simulink model "simulation"  (R2020a)
settings: Solver=VariableStepAuto  StartTime=0.0  StopTime=55  RelTol=1e-3
values from neighbouring files (symbols this model uses):
  gates = [zeros(36,1);zeros(3*length(cars)/18,1)]    [init.m]
  isReroute = 0    [init.m]
  J = 10000000    [init.m]
  rule = 1    [init.m]
  sequences = cars    [init.m]
  T = 10000000    [init.m]
  threshold = 200    [init.m]
  x0 = [reshape(areas,45,1);cars]    [init.m]
libraries: simulink x9
settings Model: Creator=Admin  LastModifiedBy=Admin

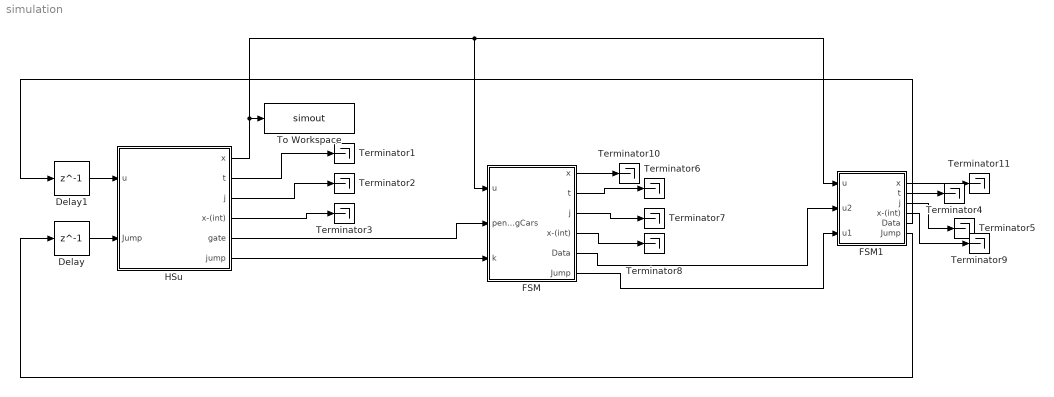
== system simulation ==
  Delay : Delay  DelayLength=1  InitialCondition=0
  Delay1 : Delay  DelayLength=1  InitialCondition=0
  FSM : Subsystem  LoadFcn=set_param(gcb,'LinkStatus','none')
      settings: CopyFcn=|
      | set_param(gcb,'LinkStatus','none'),
      | set_param(gcs, 'MaxStep', 'MaxStep', 'RelTol', 'RelTol','Stop time', 'T')
      mask Display:
      | image(imread('FSM.jpg'))
      | %plot([5 20 20 5 5],[5 5 20 20 5])
      | %text(8,13,'HyEq_mdl')
      | port_label('output', 1, 'x')
      | port_label('output', 2, 't')
      | port_label('output', 3, 'j')
      | port_label('output', 4, 'x-(int)')
      | port_label('input', 1, 'u')
  FSM1 : Subsystem  LoadFcn=set_param(gcb,'LinkStatus','none')
      settings: CopyFcn=|
      | set_param(gcb,'LinkStatus','none'),
      | set_param(gcs, 'MaxStep', 'MaxStep', 'RelTol', 'RelTol','Stop time', 'T')
      mask Display:
      | image(imread('FSM.jpg'))
      | %plot([5 20 20 5 5],[5 5 20 20 5])
      | %text(8,13,'HyEq_mdl')
      | port_label('output', 1, 'x')
      | port_label('output', 2, 't')
      | port_label('output', 3, 'j')
      | port_label('output', 4, 'x-(int)')
      | port_label('input', 1, 'u')
  HSu : Subsystem  LoadFcn=set_param(gcb,'LinkStatus','none')
      settings: CopyFcn=|
      | set_param(gcb,'LinkStatus','none'),
      | set_param(gcs, 'MaxStep', 'MaxStep', 'RelTol', 'RelTol','Stop time', 'T')
      mask Display:
      | image(imread('Cplant.jpg'))
      | %plot([5 20 20 5 5],[5 5 20 20 5])
      | %text(8,13,'HyEq_mdl')
      | port_label('output', 1, 'x')
      | port_label('output', 2, 't')
      | port_label('output', 3, 'j')
      | port_label('output', 4, 'x-(int)')
      | port_label('input', 1, 'u')
  Terminator{1..11} (11 alike) : Terminator
  To Workspace : ToWorkspace  VariableName=simout  SaveFormat=Timeseries  SampleTime=-1
  wires:
  FSM/2(t) -> Terminator6/1
  FSM/3(j) -> Terminator7/1
  FSM/4(x-(int)) -> Terminator8/1
  HSu/2(t) -> Terminator1/1
  HSu/3(j) -> Terminator2/1
  HSu/4(x-(int)) -> Terminator3/1
  FSM1/4(x-(int)) -> Terminator9/1
  FSM1/3(j) -> Terminator5/1
  FSM1/2(t) -> Terminator4/1
  HSu/6(jump) -> FSM/3(k)
  FSM/5(Data) -> FSM1/2(u2)
  HSu/5(gate) -> FSM/2(pendingCars)
  FSM/1(x) -> Terminator10/1
  FSM/6(Jump) -> FSM1/3(u1)
  FSM1/1(x) -> Terminator11/1
  FSM1/6(Jump) -> Delay/1
  FSM1/5(Data) -> Delay1/1
  HSu/1(x) -> FSM/1(u), FSM1/1(u), To Workspace/1
  Delay/1 -> HSu/2(Jump)
  Delay1/1 -> HSu/1(u)

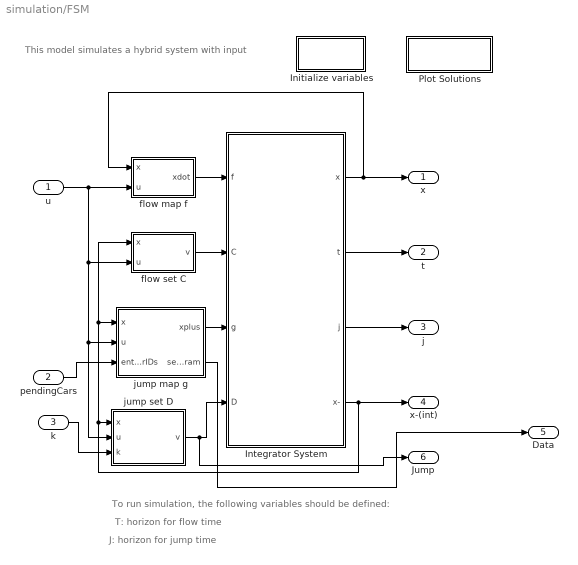
== system simulation/FSM ==
  note: J: horizon for jump time
  note: T: horizon for flow time
  note: To run simulation, the following variables should be defined:
  note: This model simulates a hybrid system with input
  u : Inport
  pendingCars : Inport  Port=2
  k : Inport  Port=3
  Initialize variables : Subsystem  Priority=-10
      settings: OpenFcn=|
      | try
      |      clearvars -except inifile pathfile_in pathfile_pos posfile
      |      cd(pathfile_in);
      |      eval(inifile);
      | catch
      |      [inifile,pathfile_in] = getInitializationfile;
      |      cd(pathfile_in);
      |      inifile = strrep(inifile,'.m','');
      |      eval(inifile);
      | end
      mask Display: disp('Double Click\n to Initialize')
  Integrator System : Subsystem  Priority=2  mask(Hybrid Integrator){T=T, J=J, x0=gates}
      mask prompts: T "Flow Horizon"; J "Jump Horizon"; x0 "Initial Condition"
      mask help:
      | This block integrates the state of the hybrid system defined by the flow map f (first input), the flow set C (second input), the jump map g (third input) and the jump set D (fourth input).
      | Starting from the initial condition x0 (last mask parameter), the system's state x evolves continuously within the set C, according to f(x,u), but is also subject to jumps within D, according to g(x,u).
      | The block also stops the simulation when the time t is greater than the flow horizon T (first mask parameter), or when the number of jumps j is greater than the jump horizon J (second mask parameter).
      | The outputs of the blocks are respectively x(t), t, j, x(t-).
      mask Help:
      | This block integrates the state of the hybrid system defined by the flow map f (first input), the flow set C (second input), the jump map g (third input) and the jump set D (fourth input).
      | <br>
      | Starting from the initial condition x0 (last mask parameter), the system's state x evolves continuously within the set C, according to f(x,u), but is also subject to jumps within D, according to g(x,u).
      | <br>
      | The block also stops the simulation when the time t is greater than the flow horizon T (first mask parameter), or when the number of jumps j is greater than the jump horizon J (second mask parameter).
      | <br>
      | The outputs of the blocks are respectively x(t), t, j, x(t-).
      | <br>
      | You can right click on the block and "Look under mask" to see what's inside the block.
      | Finally, refer to the manual (HybridSimulator_vXX.pdf) for more detailed information on how this hybrid simulator works.
  Plot Solutions : Subsystem
      settings: OpenFcn=|
      | try
      |      cd(pathfile_pos);
      |      eval(posfile);
      | catch
      |      [posfile,pathfile_pos] = getInitializationfile;
      |      cd(pathfile_pos);
      |      posfile = strrep(posfile,'.m','');
      |      eval(posfile);
      | end
      mask Display: disp('Double Click to\n Plot Solutions')
  flow map f : MATLAB Function  TreatAsAtomicUnit=on
  flow set C : MATLAB Function  TreatAsAtomicUnit=on
  jump map g : MATLAB Function  Priority=2  TreatAsAtomicUnit=on
  jump set D : MATLAB Function  TreatAsAtomicUnit=on
  x : Outport
  t : Outport  Port=2
  j : Outport  Port=3
  x-(int) : Outport  Port=4
  Data : Outport  Port=5
  Jump : Outport  Port=6
  wires:
  jump map g/1(xplus) -> Integrator System/3(g)
  jump set D/1(v) -> Jump/1, Integrator System/4(D)
  u/1 -> jump set D/2(u), jump map g/2(u), flow set C/2(u), flow map f/2(u)
  Integrator System/3(j) -> j/1
  Integrator System/2(t) -> t/1
  flow set C/1(v) -> Integrator System/2(C)
  Integrator System/1(x) -> x/1, flow map f/1(x)
  Integrator System/4(x-) -> x-(int)/1, flow set C/1(x), jump map g/1(x), jump set D/1(x)
  flow map f/1(xdot) -> Integrator System/1(f)
  pendingCars/1 -> jump map g/3(enteringCarIDs)
  k/1 -> jump set D/3(k)
  jump map g/2(seqParam) -> Data/1

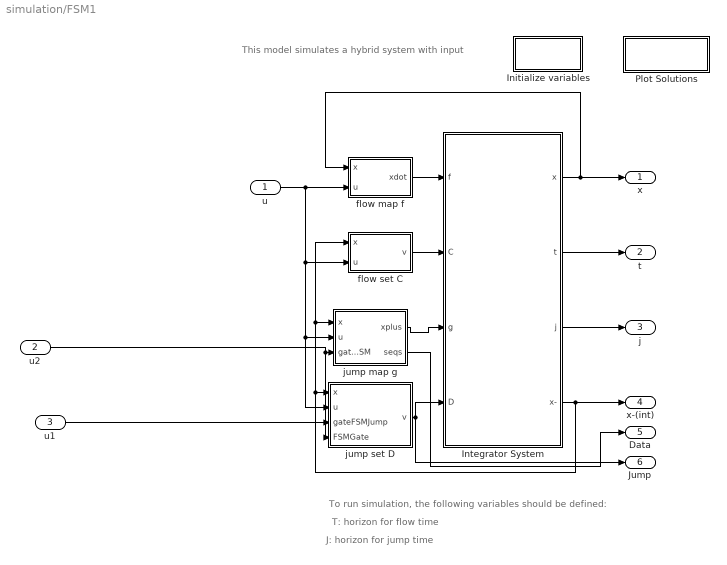
== system simulation/FSM1 ==
  note: J: horizon for jump time
  note: T: horizon for flow time
  note: To run simulation, the following variables should be defined:
  note: This model simulates a hybrid system with input
  u : Inport
  u2 : Inport  Port=2
  u1 : Inport  Port=3
  Initialize variables : Subsystem  Priority=-10
      settings: OpenFcn=|
      | try
      |      clearvars -except inifile pathfile_in pathfile_pos posfile
      |      cd(pathfile_in);
      |      eval(inifile);
      | catch
      |      [inifile,pathfile_in] = getInitializationfile;
      |      cd(pathfile_in);
      |      inifile = strrep(inifile,'.m','');
      |      eval(inifile);
      | end
      mask Display: disp('Double Click\n to Initialize')
  Integrator System : Subsystem  Priority=2  mask(Hybrid Integrator){T=T, J=J, x0=sequences}
      mask prompts: T "Flow Horizon"; J "Jump Horizon"; x0 "Initial Condition"
      mask help:
      | This block integrates the state of the hybrid system defined by the flow map f (first input), the flow set C (second input), the jump map g (third input) and the jump set D (fourth input).
      | Starting from the initial condition x0 (last mask parameter), the system's state x evolves continuously within the set C, according to f(x,u), but is also subject to jumps within D, according to g(x,u).
      | The block also stops the simulation when the time t is greater than the flow horizon T (first mask parameter), or when the number of jumps j is greater than the jump horizon J (second mask parameter).
      | The outputs of the blocks are respectively x(t), t, j, x(t-).
      mask Help:
      | This block integrates the state of the hybrid system defined by the flow map f (first input), the flow set C (second input), the jump map g (third input) and the jump set D (fourth input).
      | <br>
      | Starting from the initial condition x0 (last mask parameter), the system's state x evolves continuously within the set C, according to f(x,u), but is also subject to jumps within D, according to g(x,u).
      | <br>
      | The block also stops the simulation when the time t is greater than the flow horizon T (first mask parameter), or when the number of jumps j is greater than the jump horizon J (second mask parameter).
      | <br>
      | The outputs of the blocks are respectively x(t), t, j, x(t-).
      | <br>
      | You can right click on the block and "Look under mask" to see what's inside the block.
      | Finally, refer to the manual (HybridSimulator_vXX.pdf) for more detailed information on how this hybrid simulator works.
  Plot Solutions : Subsystem
      settings: OpenFcn=|
      | try
      |      cd(pathfile_pos);
      |      eval(posfile);
      | catch
      |      [posfile,pathfile_pos] = getInitializationfile;
      |      cd(pathfile_pos);
      |      posfile = strrep(posfile,'.m','');
      |      eval(posfile);
      | end
      mask Display: disp('Double Click to\n Plot Solutions')
  flow map f : MATLAB Function  TreatAsAtomicUnit=on
  flow set C : MATLAB Function  TreatAsAtomicUnit=on
  jump map g : MATLAB Function  Priority=2  TreatAsAtomicUnit=on
  jump set D : MATLAB Function  TreatAsAtomicUnit=on
  x : Outport
  t : Outport  Port=2
  j : Outport  Port=3
  x-(int) : Outport  Port=4
  Data : Outport  Port=5
  Jump : Outport  Port=6
  wires:
  jump map g/1(xplus) -> Integrator System/3(g)
  jump set D/1(v) -> Integrator System/4(D), Jump/1
  u/1 -> jump set D/2(u), jump map g/2(u), flow set C/2(u), flow map f/2(u)
  Integrator System/3(j) -> j/1
  Integrator System/2(t) -> t/1
  flow set C/1(v) -> Integrator System/2(C)
  Integrator System/1(x) -> x/1, flow map f/1(x)
  Integrator System/4(x-) -> x-(int)/1, flow set C/1(x), jump map g/1(x), jump set D/1(x)
  flow map f/1(xdot) -> Integrator System/1(f)
  u2/1 -> jump set D/4(FSMGate), jump map g/3(gateFSM)
  u1/1 -> jump set D/3(gateFSMJump)
  jump map g/2(seqs) -> Data/1

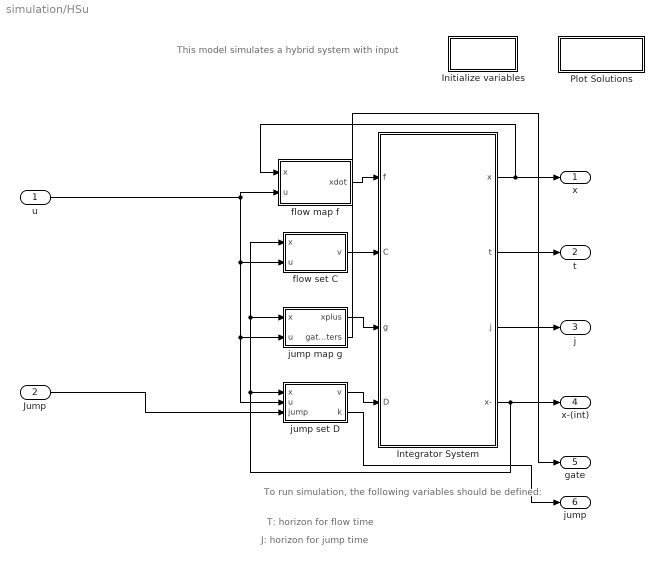
== system simulation/HSu ==
  note: J: horizon for jump time
  note: T: horizon for flow time
  note: To run simulation, the following variables should be defined:
  note: This model simulates a hybrid system with input
  u : Inport
  Jump : Inport  Port=2
  Initialize variables : Subsystem  Priority=-10
      settings: OpenFcn=|
      | try
      |      clearvars -except inifile pathfile_in pathfile_pos posfile
      |      cd(pathfile_in);
      |      eval(inifile);
      | catch
      |      [inifile,pathfile_in] = getInitializationfile;
      |      cd(pathfile_in);
      |      inifile = strrep(inifile,'.m','');
      |      eval(inifile);
      | end
      mask Display: disp('Double Click\n to Initialize')
  Integrator System : Subsystem  Priority=2  mask(Hybrid Integrator){T=T, J=J, x0=x0}
      mask prompts: T "Flow Horizon"; J "Jump Horizon"; x0 "Initial Condition"
      mask help:
      | This block integrates the state of the hybrid system defined by the flow map f (first input), the flow set C (second input), the jump map g (third input) and the jump set D (fourth input).
      | Starting from the initial condition x0 (last mask parameter), the system's state x evolves continuously within the set C, according to f(x,u), but is also subject to jumps within D, according to g(x,u).
      | The block also stops the simulation when the time t is greater than the flow horizon T (first mask parameter), or when the number of jumps j is greater than the jump horizon J (second mask parameter).
      | The outputs of the blocks are respectively x(t), t, j, x(t-).
      mask Help:
      | This block integrates the state of the hybrid system defined by the flow map f (first input), the flow set C (second input), the jump map g (third input) and the jump set D (fourth input).
      | <br>
      | Starting from the initial condition x0 (last mask parameter), the system's state x evolves continuously within the set C, according to f(x,u), but is also subject to jumps within D, according to g(x,u).
      | <br>
      | The block also stops the simulation when the time t is greater than the flow horizon T (first mask parameter), or when the number of jumps j is greater than the jump horizon J (second mask parameter).
      | <br>
      | The outputs of the blocks are respectively x(t), t, j, x(t-).
      | <br>
      | You can right click on the block and "Look under mask" to see what's inside the block.
      | Finally, refer to the manual (HybridSimulator_vXX.pdf) for more detailed information on how this hybrid simulator works.
  Plot Solutions : Subsystem
      settings: OpenFcn=|
      | try
      |      cd(pathfile_pos);
      |      eval(posfile);
      | catch
      |      [posfile,pathfile_pos] = getInitializationfile;
      |      cd(pathfile_pos);
      |      posfile = strrep(posfile,'.m','');
      |      eval(posfile);
      | end
      mask Display: disp('Double Click to\n Plot Solutions')
  flow map f : MATLAB Function  TreatAsAtomicUnit=on
  flow set C : MATLAB Function  TreatAsAtomicUnit=on
  jump map g : MATLAB Function  Priority=2  TreatAsAtomicUnit=on
  jump set D : MATLAB Function  TreatAsAtomicUnit=on
  x : Outport
  t : Outport  Port=2
  j : Outport  Port=3
  x-(int) : Outport  Port=4
  gate : Outport  Port=5
  jump : Outport  Port=6
  wires:
  jump map g/1(xplus) -> Integrator System/3(g)
  jump set D/1(v) -> Integrator System/4(D)
  u/1 -> jump set D/2(u), jump map g/2(u), flow set C/2(u), flow map f/2(u)
  Integrator System/3(j) -> j/1
  Integrator System/2(t) -> t/1
  flow set C/1(v) -> Integrator System/2(C)
  Integrator System/1(x) -> x/1, flow map f/1(x)
  Integrator System/4(x-) -> x-(int)/1, jump set D/1(x), flow set C/1(x), jump map g/1(x)
  flow map f/1(xdot) -> Integrator System/1(f)
  jump map g/2(gateParameters) -> gate/1
  jump set D/2(k) -> jump/1
  Jump/1 -> jump set D/3(jump)

== system simulation/FSM/Initialize variables ==

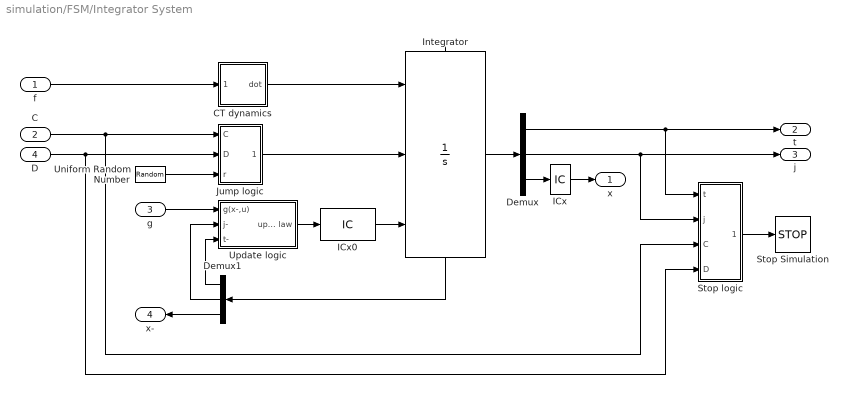
== system simulation/FSM/Integrator System ==
  f : Inport
  C : Inport  Port=2
  g : Inport  Port=3
  D : Inport  Port=4
  CT dynamics : Subsystem
  Demux : Demux  Outputs=[1 1 -1]
  Demux1 : Demux  Outputs=[1 1 -1]
  ICx : InitialCondition  Value=x0
  ICx0 : InitialCondition  Value=[0; 0; x0(:)]
  Integrator : Integrator  ExternalReset=level hold  InitialConditionSource=external  ShowStatePort=on  ZeroCross=off
  Jump logic : Subsystem
  Stop Simulation : Stop
  Stop logic : Subsystem
  Uniform Random Number : UniformRandomNumber  Minimum=0  Seed=abs(floor(100*rand))  SampleTime=0
  Update logic : Subsystem
  x : Outport
  t : Outport  Port=2
  j : Outport  Port=3
  x- : Outport  Port=4
  wires:
  ICx0/1 -> Integrator/3
  ICx/1 -> x/1
  Demux/3 -> ICx/1
  Integrator/State -> Demux1/1
  Demux/2 -> j/1, Stop logic/2(j)
  Demux/1 -> t/1, Stop logic/1(t)
  Update logic/1(update law) -> ICx0/1
  CT dynamics/1(dot) -> Integrator/1
  Stop logic/1(stop) -> Stop Simulation/1
  Integrator/1 -> Demux/1
  C/1 -> Stop logic/3(C), Jump logic/1(C)
  D/1 -> Stop logic/4(D), Jump logic/2(D)
  f/1 -> CT dynamics/1(f(x,u))
  Demux1/3 -> x-/1
  Jump logic/1(jump) -> Integrator/2
  Uniform Random Number/1 -> Jump logic/3(r)
  g/1 -> Update logic/1(g(x-,u))
  Demux1/1 -> Update logic/3(t-)
  Demux1/2 -> Update logic/2(j-)

== system simulation/FSM/Plot Solutions ==

== system simulation/FSM1/Initialize variables ==

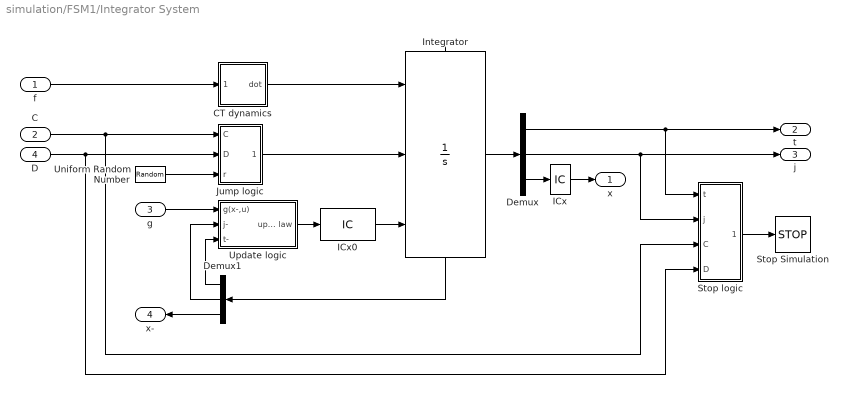
== system simulation/FSM1/Integrator System ==
  f : Inport
  C : Inport  Port=2
  g : Inport  Port=3
  D : Inport  Port=4
  CT dynamics : Subsystem
  Demux : Demux  Outputs=[1 1 -1]
  Demux1 : Demux  Outputs=[1 1 -1]
  ICx : InitialCondition  Value=x0
  ICx0 : InitialCondition  Value=[0; 0; x0(:)]
  Integrator : Integrator  ExternalReset=level hold  InitialConditionSource=external  ShowStatePort=on  ZeroCross=off
  Jump logic : Subsystem
  Stop Simulation : Stop
  Stop logic : Subsystem
  Uniform Random Number : UniformRandomNumber  Minimum=0  Seed=abs(floor(100*rand))  SampleTime=0
  Update logic : Subsystem
  x : Outport
  t : Outport  Port=2
  j : Outport  Port=3
  x- : Outport  Port=4
  wires:
  ICx0/1 -> Integrator/3
  ICx/1 -> x/1
  Demux/3 -> ICx/1
  Integrator/State -> Demux1/1
  Demux/2 -> j/1, Stop logic/2(j)
  Demux/1 -> t/1, Stop logic/1(t)
  Update logic/1(update law) -> ICx0/1
  CT dynamics/1(dot) -> Integrator/1
  Stop logic/1(stop) -> Stop Simulation/1
  Integrator/1 -> Demux/1
  C/1 -> Stop logic/3(C), Jump logic/1(C)
  D/1 -> Stop logic/4(D), Jump logic/2(D)
  f/1 -> CT dynamics/1(f(x,u))
  Demux1/3 -> x-/1
  Jump logic/1(jump) -> Integrator/2
  Uniform Random Number/1 -> Jump logic/3(r)
  g/1 -> Update logic/1(g(x-,u))
  Demux1/1 -> Update logic/3(t-)
  Demux1/2 -> Update logic/2(j-)

== system simulation/FSM1/Plot Solutions ==

== system simulation/HSu/Initialize variables ==

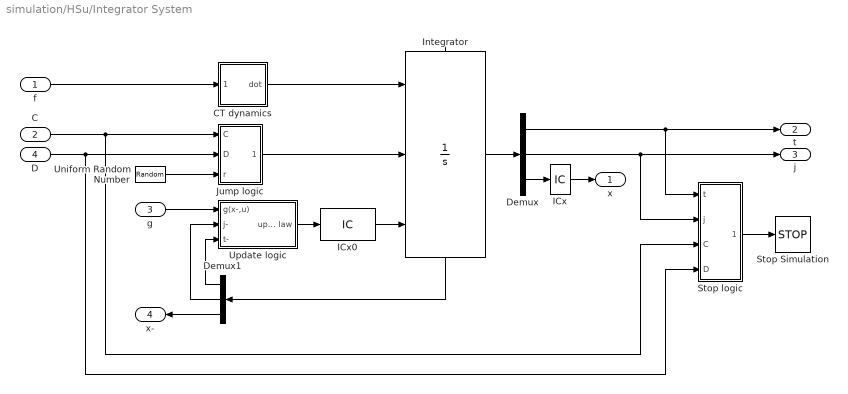
== system simulation/HSu/Integrator System ==
  f : Inport
  C : Inport  Port=2
  g : Inport  Port=3
  D : Inport  Port=4
  CT dynamics : Subsystem
  Demux : Demux  Outputs=[1 1 -1]
  Demux1 : Demux  Outputs=[1 1 -1]
  ICx : InitialCondition  Value=x0
  ICx0 : InitialCondition  Value=[0; 0; x0(:)]
  Integrator : Integrator  ExternalReset=level hold  InitialConditionSource=external  ShowStatePort=on  ZeroCross=off
  Jump logic : Subsystem
  Stop Simulation : Stop
  Stop logic : Subsystem
  Uniform Random Number : UniformRandomNumber  Minimum=0  Seed=abs(floor(100*rand))  SampleTime=0
  Update logic : Subsystem
  x : Outport
  t : Outport  Port=2
  j : Outport  Port=3
  x- : Outport  Port=4
  wires:
  ICx0/1 -> Integrator/3
  ICx/1 -> x/1
  Demux/3 -> ICx/1
  Integrator/State -> Demux1/1
  Demux/2 -> j/1, Stop logic/2(j)
  Demux/1 -> t/1, Stop logic/1(t)
  Update logic/1(update law) -> ICx0/1
  CT dynamics/1(dot) -> Integrator/1
  Stop logic/1(stop) -> Stop Simulation/1
  Integrator/1 -> Demux/1
  C/1 -> Stop logic/3(C), Jump logic/1(C)
  D/1 -> Stop logic/4(D), Jump logic/2(D)
  f/1 -> CT dynamics/1(f(x,u))
  Demux1/3 -> x-/1
  Jump logic/1(jump) -> Integrator/2
  Uniform Random Number/1 -> Jump logic/3(r)
  g/1 -> Update logic/1(g(x-,u))
  Demux1/1 -> Update logic/3(t-)
  Demux1/2 -> Update logic/2(j-)

== system simulation/HSu/Plot Solutions ==

== system simulation/FSM/Integrator System/CT dynamics ==
  f(x,u) : Inport
  Flows : Constant
  Jumps : Constant  Value=0
  Mux : Mux  Inputs=[1 1 -1]
  dot : Outport
  wires:
  Jumps/1 -> Mux/2
  Flows/1 -> Mux/1
  Mux/1 -> dot/1
  f(x,u)/1 -> Mux/3

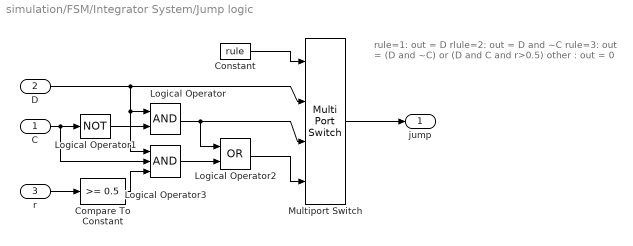
== system simulation/FSM/Integrator System/Jump logic ==
  note: rule=1:  out = D
      | rlule=2: out = D and ~C
      | rule=3:  out = (D and ~C)  or (D and C and r>0.5)
      | other :  out = 0
  C : Inport
  D : Inport  Port=2
  r : Inport  Port=3
  Compare To Constant : simulink/Logic and Bit Operations/Compare To Constant  relop=>=  const=0.5  OutDataTypeStr=uint8
  Constant : Constant  Value=rule
  Logical Operator : Logic  AllPortsSameDT=off  OutDataTypeStr=boolean
  Logical Operator1 : Logic  Operator=NOT  Inputs=1  AllPortsSameDT=off  OutDataTypeStr=boolean
  Logical Operator2 : Logic  Operator=OR  AllPortsSameDT=off  OutDataTypeStr=boolean
  Logical Operator3 : Logic  Inputs=3  AllPortsSameDT=off  OutDataTypeStr=boolean
  Multiport Switch : MultiPortSwitch
  jump : Outport
  wires:
  Constant/1 -> Multiport Switch/1
  D/1 -> Logical Operator3/1, Logical Operator/1, Multiport Switch/2
  r/1 -> Compare To Constant/1
  C/1 -> Logical Operator3/2, Logical Operator1/1
  Logical Operator1/1 -> Logical Operator/2
  Logical Operator/1 -> Multiport Switch/3, Logical Operator2/1
  Logical Operator2/1 -> Multiport Switch/4
  Multiport Switch/1 -> jump/1
  Compare To Constant/1 -> Logical Operator3/3
  Logical Operator3/1 -> Logical Operator2/2

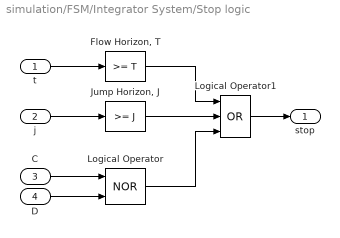
== system simulation/FSM/Integrator System/Stop logic ==
  t : Inport
  j : Inport  Port=2
  C : Inport  Port=3
  D : Inport  Port=4
  "Flow Horizon, T" : simulink/Logic and Bit Operations/Compare To Constant  relop=>=  const=T  OutDataTypeStr=uint8  ZeroCross=off
  "Jump Horizon, J" : simulink/Logic and Bit Operations/Compare To Constant  relop=>=  const=J  OutDataTypeStr=uint8  ZeroCross=off
  Logical Operator : Logic  Operator=NOR  AllPortsSameDT=off  OutDataTypeStr=boolean
  Logical Operator1 : Logic  Operator=OR  Inputs=3  AllPortsSameDT=off  OutDataTypeStr=boolean
  stop : Outport
  wires:
  "Flow Horizon, T"/1 -> Logical Operator1/1
  "Jump Horizon, J"/1 -> Logical Operator1/2
  Logical Operator/1 -> Logical Operator1/3
  D/1 -> Logical Operator/2
  t/1 -> "Flow Horizon, T"/1
  j/1 -> "Jump Horizon, J"/1
  C/1 -> Logical Operator/1
  Logical Operator1/1 -> stop/1

== system simulation/FSM/Integrator System/Update logic ==
  g(x-,u) : Inport
  j- : Inport  Port=2
  t- : Inport  Port=3
  Constant : Constant
  Mux1 : Mux  Inputs=[1 1 -1]
  Sum : Sum  Inputs=|++
  update law : Outport
  wires:
  Sum/1 -> Mux1/2
  Mux1/1 -> update law/1
  j-/1 -> Sum/1
  g(x-,u)/1 -> Mux1/3
  t-/1 -> Mux1/1
  Constant/1 -> Sum/2

== system simulation/FSM1/Integrator System/CT dynamics ==
  f(x,u) : Inport
  Flows : Constant
  Jumps : Constant  Value=0
  Mux : Mux  Inputs=[1 1 -1]
  dot : Outport
  wires:
  Jumps/1 -> Mux/2
  Flows/1 -> Mux/1
  Mux/1 -> dot/1
  f(x,u)/1 -> Mux/3

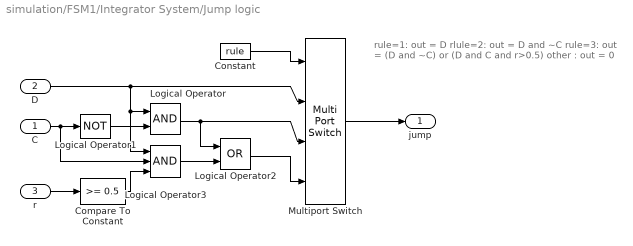
== system simulation/FSM1/Integrator System/Jump logic ==
  note: rule=1:  out = D
      | rlule=2: out = D and ~C
      | rule=3:  out = (D and ~C)  or (D and C and r>0.5)
      | other :  out = 0
  C : Inport
  D : Inport  Port=2
  r : Inport  Port=3
  Compare To Constant : simulink/Logic and Bit Operations/Compare To Constant  relop=>=  const=0.5  OutDataTypeStr=uint8
  Constant : Constant  Value=rule
  Logical Operator : Logic  AllPortsSameDT=off  OutDataTypeStr=boolean
  Logical Operator1 : Logic  Operator=NOT  Inputs=1  AllPortsSameDT=off  OutDataTypeStr=boolean
  Logical Operator2 : Logic  Operator=OR  AllPortsSameDT=off  OutDataTypeStr=boolean
  Logical Operator3 : Logic  Inputs=3  AllPortsSameDT=off  OutDataTypeStr=boolean
  Multiport Switch : MultiPortSwitch
  jump : Outport
  wires:
  Constant/1 -> Multiport Switch/1
  D/1 -> Logical Operator3/1, Logical Operator/1, Multiport Switch/2
  r/1 -> Compare To Constant/1
  C/1 -> Logical Operator3/2, Logical Operator1/1
  Logical Operator1/1 -> Logical Operator/2
  Logical Operator/1 -> Multiport Switch/3, Logical Operator2/1
  Logical Operator2/1 -> Multiport Switch/4
  Multiport Switch/1 -> jump/1
  Compare To Constant/1 -> Logical Operator3/3
  Logical Operator3/1 -> Logical Operator2/2

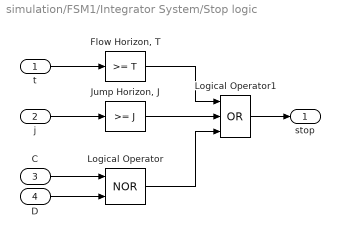
== system simulation/FSM1/Integrator System/Stop logic ==
  t : Inport
  j : Inport  Port=2
  C : Inport  Port=3
  D : Inport  Port=4
  "Flow Horizon, T" : simulink/Logic and Bit Operations/Compare To Constant  relop=>=  const=T  OutDataTypeStr=uint8  ZeroCross=off
  "Jump Horizon, J" : simulink/Logic and Bit Operations/Compare To Constant  relop=>=  const=J  OutDataTypeStr=uint8  ZeroCross=off
  Logical Operator : Logic  Operator=NOR  AllPortsSameDT=off  OutDataTypeStr=boolean
  Logical Operator1 : Logic  Operator=OR  Inputs=3  AllPortsSameDT=off  OutDataTypeStr=boolean
  stop : Outport
  wires:
  "Flow Horizon, T"/1 -> Logical Operator1/1
  "Jump Horizon, J"/1 -> Logical Operator1/2
  Logical Operator/1 -> Logical Operator1/3
  D/1 -> Logical Operator/2
  t/1 -> "Flow Horizon, T"/1
  j/1 -> "Jump Horizon, J"/1
  C/1 -> Logical Operator/1
  Logical Operator1/1 -> stop/1

== system simulation/FSM1/Integrator System/Update logic ==
  g(x-,u) : Inport
  j- : Inport  Port=2
  t- : Inport  Port=3
  Constant : Constant
  Mux1 : Mux  Inputs=[1 1 -1]
  Sum : Sum  Inputs=|++
  update law : Outport
  wires:
  Sum/1 -> Mux1/2
  Mux1/1 -> update law/1
  j-/1 -> Sum/1
  g(x-,u)/1 -> Mux1/3
  t-/1 -> Mux1/1
  Constant/1 -> Sum/2

== system simulation/HSu/Integrator System/CT dynamics ==
  f(x,u) : Inport
  Flows : Constant
  Jumps : Constant  Value=0
  Mux : Mux  Inputs=[1 1 -1]
  dot : Outport
  wires:
  Jumps/1 -> Mux/2
  Flows/1 -> Mux/1
  Mux/1 -> dot/1
  f(x,u)/1 -> Mux/3

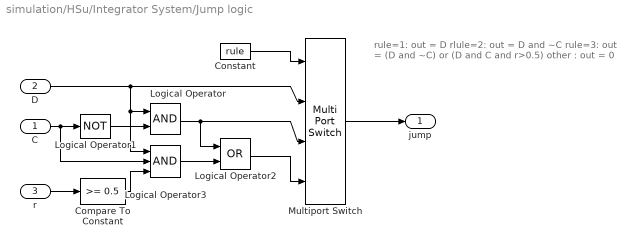
== system simulation/HSu/Integrator System/Jump logic ==
  note: rule=1:  out = D
      | rlule=2: out = D and ~C
      | rule=3:  out = (D and ~C)  or (D and C and r>0.5)
      | other :  out = 0
  C : Inport
  D : Inport  Port=2
  r : Inport  Port=3
  Compare To Constant : simulink/Logic and Bit Operations/Compare To Constant  relop=>=  const=0.5  OutDataTypeStr=uint8
  Constant : Constant  Value=rule
  Logical Operator : Logic  AllPortsSameDT=off  OutDataTypeStr=boolean
  Logical Operator1 : Logic  Operator=NOT  Inputs=1  AllPortsSameDT=off  OutDataTypeStr=boolean
  Logical Operator2 : Logic  Operator=OR  AllPortsSameDT=off  OutDataTypeStr=boolean
  Logical Operator3 : Logic  Inputs=3  AllPortsSameDT=off  OutDataTypeStr=boolean
  Multiport Switch : MultiPortSwitch
  jump : Outport
  wires:
  Constant/1 -> Multiport Switch/1
  D/1 -> Logical Operator3/1, Logical Operator/1, Multiport Switch/2
  r/1 -> Compare To Constant/1
  C/1 -> Logical Operator3/2, Logical Operator1/1
  Logical Operator1/1 -> Logical Operator/2
  Logical Operator/1 -> Multiport Switch/3, Logical Operator2/1
  Logical Operator2/1 -> Multiport Switch/4
  Multiport Switch/1 -> jump/1
  Compare To Constant/1 -> Logical Operator3/3
  Logical Operator3/1 -> Logical Operator2/2

== system simulation/HSu/Integrator System/Stop logic ==
  t : Inport
  j : Inport  Port=2
  C : Inport  Port=3
  D : Inport  Port=4
  "Flow Horizon, T" : simulink/Logic and Bit Operations/Compare To Constant  relop=>=  const=T  OutDataTypeStr=uint8  ZeroCross=off
  "Jump Horizon, J" : simulink/Logic and Bit Operations/Compare To Constant  relop=>=  const=J  OutDataTypeStr=uint8  ZeroCross=off
  Logical Operator : Logic  Operator=NOR  AllPortsSameDT=off  OutDataTypeStr=boolean
  Logical Operator1 : Logic  Operator=OR  Inputs=3  AllPortsSameDT=off  OutDataTypeStr=boolean
  stop : Outport
  wires:
  "Flow Horizon, T"/1 -> Logical Operator1/1
  "Jump Horizon, J"/1 -> Logical Operator1/2
  Logical Operator/1 -> Logical Operator1/3
  D/1 -> Logical Operator/2
  t/1 -> "Flow Horizon, T"/1
  j/1 -> "Jump Horizon, J"/1
  C/1 -> Logical Operator/1
  Logical Operator1/1 -> stop/1

== system simulation/HSu/Integrator System/Update logic ==
  g(x-,u) : Inport
  j- : Inport  Port=2
  t- : Inport  Port=3
  Constant : Constant
  Mux1 : Mux  Inputs=[1 1 -1]
  Sum : Sum  Inputs=|++
  update law : Outport
  wires:
  Sum/1 -> Mux1/2
  Mux1/1 -> update law/1
  j-/1 -> Sum/1
  g(x-,u)/1 -> Mux1/3
  t-/1 -> Mux1/1
  Constant/1 -> Sum/2

== matlab function simulation/HSu/flow set C ==
  data: x input; v output; u input
function v  = C(x, u) 
%--------------------------------------------------------------------------
% Matlab M-file Project: HyEQ Toolbox @  Hybrid Systems Laboratory (HSL), 
% https://hybrid.soe.ucsc.edu/software
% http://hybridsimulator.wordpress.com/
%--------------------------------------------------------------------------
% Project: Simulation of a hybrid system
% Description: Flow set
%--------------------------------------------------------------------------
%--------------------------------------------------------------------------
%   See also HYEQSOLVER, PLOTARC, PLOTARC3, PLOTFLOWS, PLOTHARC,
%   PLOTHARCCOLOR, PLOTHARCCOLOR3D, PLOTHYBRIDARC, PLOTJUMPS.
%   Copyright @ Hybrid Systems Laboratory (HSL),
%   Revision: 0.0.0.3 Date: 05/20/2015 3:42:00
%
% Check on flow conditions
% E.g.,
% if (x(1) >= u(1))  % flow condition
%     v = 1;  % report flow
% else
%     v = 0;   % do not report flow
% end

    v = 1; % report flow

end

== matlab function simulation/HSu/jump map g ==
  settings: updateMethod=DISCRETE
  data: x input; xplus output; u input; gateParameters output
function [xplus,gateParameters]= g(x, u)

cars = x(46:end);
carMatrix = reshape(cars,length(cars)/18,18);

% admittedCarMatrix = reshape(u,3,length(u)/3)';
admittedCarMatrix = u;
% newCarMatrix = carMatrix;

% for i =1:length(cars)/18
%     if isequal(carMatrix(i,[9,10]),newCarMatrix(i,[9,10]))
%         admittedCars=[admittedCars,i];
%     end
% end
for i = 1:length(cars)/18
    if admittedCarMatrix(i,1)~=carMatrix(i,17)
        
        carMatrix(i,[17,9,10,11]) = admittedCarMatrix(i,:);
        carMatrix(i,13)=1;
        carMatrix(i,14)=0;
    end
end


carPlus=zeros(length(cars)/18,18);
gateParameters = zeros(length(cars)/18,1);


for i = 1:length(cars)/18
    [carPlus(i,:),RFID] =carJumpC(carMatrix(i,:));
   
    if RFID>0
        gateParameters(RFID)=1;
    end
end
 
carPlus=reshape(carPlus,length(cars),1);
areaMatrix = reshape(x(1:45),9,5);
xplus = [reshape(areaMatrix,45,1);carPlus];
end

== matlab function simulation/HSu/jump set D ==
  data: x input; v output; u input; k output; jump input
function [v,k] = D(x, u,jump) 

cars = x(46:end);
% 
carMatrix = reshape(cars,length(cars)/18,18);
% newCarMatrix = reshape(u,18,length(u)/18)';
v=jump==1;
% for i =1:length(cars)/18
%     if ~isequal(carMatrix(i,[9,10]),newCarMatrix(i,[9,10])) && carMatrix(i,14)==0
%         v=1;
%         break;
%     end
% end
%         

% %To Do


  for i = 1:length(cars)/18
      if v || carJumpD(carMatrix(i,:)) 
          v=1==1;
      end
  end    
 
 k = 0;
 for i =1:length(cars)/18
     if abs(carMatrix(i,7) - carMatrix(i,9))<0.15   && abs(carMatrix(i,8) - carMatrix(i,10))<0.15 && carMatrix(i,14)~=0
         k=1;
         break;
     end
 end
 
% Undeterministic_horn = rand(1)>0.9;
% v=(Deterministic) || Undeterministic_horn;
% end

== matlab function simulation/FSM1/flow map f ==
  data: x input; xdot output; u input
function xdot = f(x, u)
%--------------------------------------------------------------------------
% Matlab M-file Project: HyEQ Toolbox @  Hybrid Systems Laboratory (HSL), 
% https://hybrid.soe.ucsc.edu/software
% http://hybridsimulator.wordpress.com/
%--------------------------------------------------------------------------
% Project: Simulation of a hybrid system Finite state machine (FSM)
% Description: Flow map
%--------------------------------------------------------------------------
%--------------------------------------------------------------------------
%   See also HYEQSOLVER, PLOTARC, PLOTARC3, PLOTFLOWS, PLOTHARC,
%   PLOTHARCCOLOR, PLOTHARCCOLOR3D, PLOTHYBRIDARC, PLOTJUMPS.
%   Copyright @ Hybrid Systems Laboratory (HSL),
%   Revision: 0.0.0.3 Date: 05/20/2015 3:42:00
%--------------------------------------------------------------------------
% flow map: xdot=f(x,u);

xdot =u(46:end)-x;

== matlab function simulation/FSM1/flow set C ==
  data: x input; v output; u input
function v  = C(x, u) 
%--------------------------------------------------------------------------
% Matlab M-file Project: HyEQ Toolbox @  Hybrid Systems Laboratory (HSL), 
% https://hybrid.soe.ucsc.edu/software
% http://hybridsimulator.wordpress.com/
%--------------------------------------------------------------------------
% Project: Simulation of a hybrid system Finite state machine (FSM)
% Description: Flow set
%--------------------------------------------------------------------------
%--------------------------------------------------------------------------
%   See also HYEQSOLVER, PLOTARC, PLOTARC3, PLOTFLOWS, PLOTHARC,
%   PLOTHARCCOLOR, PLOTHARCCOLOR3D, PLOTHYBRIDARC, PLOTJUMPS.
%   Copyright @ Hybrid Systems Laboratory (HSL),
%   Revision: 0.0.0.3 Date: 05/20/2015 3:42:00
%
% Check on flow conditions
% E.g.,
% if (x(1) >= u(1))  % flow condition
%     v = 1;  % report flow
% else
%     v = 0;   % do not report flow
% end

v = 1;

== matlab function simulation/FSM1/jump map g ==
  data: x input; xplus output; u input; gateFSM input; seqs output
function [xplus,seqs] = g(x, u,gateFSM)

cars = u(46:end);
carMatrix = reshape(cars,length(cars)/18,18);

carsAdmitted = gateFSM(1:length(cars)/18);
% newRouteMatrix = gateFSM(length(cars)/18 +1:end);

% newRouteMatrix = reshape(newRouteMatrix,length(cars)/18,2);
IDsRoute=zeros(length(cars)/18,1);

[carMatrixAdmit,IDsAdmit] = handleAdmit(carsAdmitted,carMatrix);

%  if isReroute==1
%      [carMatrixRoute,IDsRoute] = handleNewRoute(newRouteMatrix,carMatrix);
%  end

% carMatrix(IDsRoute==1,:)=carMatrixRoute(IDsRoute,:);

for i=1:length(IDsAdmit)
    if IDsAdmit(i)==1
        carMatrix(i,:)=carMatrixAdmit(i,:);
        carMatrix(i,[16,14])=[1,0];
    end
%     if IDsRoute(i)==1
%          carMatrix(i,:)=carMatrixRoute(i,:);
%         carMatrix(i,[16,14])=[1,0];
%     end
end

% for i=1:length(IDsAdmit)
%     if IDsAdmit(i)==1
%         carMatrix(i,:)=carMatrixAdmit(i,:);
%     end
% end

xplus = reshape(carMatrix,length(cars),1);
seqs=carMatrix(:,[17,9,10,11]);

% xplus=cars;

== matlab function simulation/FSM1/jump set D ==
  data: x input; v output; u input; gateFSMJump input; FSMGate input
function v  = D(x, u,gateFSMJump,FSMGate) 


v=1==0;
[height,width]=size(u);
if (gateFSMJump==1)&&~isequal(zeros(height,width),FSMGate)
    v=1==1;
end

== matlab function simulation/FSM/flow map f ==
  data: x input; xdot output; u input
function xdot = f(x, u)

% tmp = x(end-2);
% gateQueues = x(1:36);
% newCarAttributes = x(37:end);
% 
% gateQueueDot = zeros(length(gateQueues),1);
% newCarAttributesDot = -1.*newCarAttributes;
% xdot = [gateQueueDot;newCarAttributesDot];
xdot=zeros(length(x),1);

== matlab function simulation/FSM/flow set C ==
  data: x input; v output; u input
function v  = C(x, u) 


v = 1;

== matlab function simulation/FSM/jump map g ==
  data: x input; xplus output; u input; enteringCarIDs input; threshold parameter; isReroute parameter; seqParam output
function [xplus,seqParam] = g(x, u,enteringCarIDs,threshold,isReroute)   

gateIndex=0;
tmp = enteringCarIDs;
x2=x(1:36);

areas = u(1:45);
cars = u(46:end);

areaMatrix = reshape(areas,9,5);
carMatrix = reshape(cars,length(cars)/18,18);

carAttributes=carMatrix(:,[18,2]);

areas = reshape(areaMatrix(:,[5,1]),18,1);
areas=reshape(areas(1:18),9,2);

admittedCarIDs = zeros(length(cars)/18,1);
newRouteMatrix = zeros(length(cars)/18,2);

enteringCars = zeros(length(cars)/18,7);

carPollutions = carMatrix(:,2);

% disp(length(enteringCarIDs));

for i = 1:length(enteringCarIDs)
    if enteringCarIDs(i)==1
        enteringCars(i,:) = carMatrix(i,[1,18,5,6,11,7,8]);
        
    end
end

areaBoundaries = [-1.5,1.5,-0.5,0.5;-0.5,1.5,0.5,0.5;0.5,1.5,1.5,0.5;-1.5,0.5,-0.5,-0.5;-0.5,0.5,0.5,-0.5;0.5,0.5,1.5,-0.5;-1.5,-0.5,-0.5,-1.5;-0.5,-0.5,0.5,-1.5;0.5,-0.5,1.5,-1.5];
gatePoints = [100,100,100,100,-0.5,1,-1,0.5;
              -0.5,1,100,100,0.5,1,0,0.5;
              0.5,1,100,100,100,100,1,0.5;
            100,100,-1,0.5,-0.5,0,-1,-0.5;
            -0.5,0,0,0.5,0.5,0,0,-0.5;
            0.5,0,1,0.5,100,100,1,-0.5;
            100,100,-1,-0.5,-0.5,-1,100,100;
            -0.5,-1,0,-0.5,0.5,-1,100,100;
            0.5,-1,1,-0.5,100,100,100,100];
gateDirections = [0,0,2,4;1,0,3,5;2,0,0,6;0,1,5,7;4,2,6,8;5,3,0,9;0,4,8,0;7,5,9,0;8,6,0,0];



newGateQueue = 0;
gateQueue = 0;

for i = 1:length(enteringCarIDs)
    if enteringCarIDs(i)==0
        continue;
    end
   
    enteringCar=enteringCars(i,:);
    currArea=enteringCar(5);
    currLocation = enteringCar([6,7]);
%     Search in gate points:
    
    
    for j = 1:4
        if sum(gatePoints(currArea,[j*2-1,j*2])-reshape(currLocation,1,2))<0.15
            gateIndex=j;
        end
    end
    if gateIndex >0
        enteringArea=areas(gateDirections(currArea,gateIndex),:);
        [newGateQueue,newRoute]=enqueueGate(areaBoundaries(currArea,:),gateIndex,reshape(gatePoints(currArea,:),2,4)',x2(gateIndex) ,carPollutions,enteringCar,enteringArea,threshold,isReroute);
        if ~isequal(newRoute,[0,0])
            newRouteMatrix(i,:) = [newRoute(1),newRoute(2)];
        end

        x2(i)=newGateQueue;
    end
  
end
for i = 1:9
    for j =1:4
         gateQueue = x2((i-1)*4+j);
         if gateQueue ==0
             continue;
         end
         [admittedCar,newGateQueue] = dequeueGate(gateQueue,carAttributes,areas(i,:),threshold);
           
         x2((i-1)*4+j) = newGateQueue;
         if admittedCar >-1
             tmp = admittedCar;
             
             admittedCarIDs(admittedCar) = 1;
             
         end
    end
end
% xplus = [x2;0;0;0];
newRouteMatrix =reshape(newRouteMatrix,length(cars)/9,1);
 xplus = [x2;admittedCarIDs;newRouteMatrix];
 seqParam=[admittedCarIDs;newRouteMatrix];

== matlab function simulation/FSM/jump set D ==
  data: x input; v output; u input; k input
function v  = D(x, u,k) 
v = k==1;
% v=0;
% cars = x(46:end);
% carMatrix = reshape(cars,length(cars)/18,18);
% % if ~isempty(u)
%     newCarMatrix = reshape(u,length(u)/18,18);
% 
% 
%     for i =1:length(cars)/18
%         if isequal(carMatrix(i,[9,10]),newCarMatrix(i,[9,10])) && carMatrix(i,16)==0
%             v=1;
%             break;
%         end
%     end
% % end

== matlab function simulation/HSu/flow map f ==
  settings: updateMethod=DISCRETE
  data: x input; xdot output; u input
function xdot = f(x, u)

weather = [0.5,0.2];
areas = x(1:45);
cars = x(46:end);

areaMatrix = reshape(areas,9,5);
carMatrix = reshape(cars,length(cars)/18,18);

neighboring= [2,4,0,0;1,3,5,0;2,6,0,0;1,5,7,0;2,4,6,8;3,5,9,0;4,8,0,0;5,7,9,0;8,6,0,0;];
dissipations = getDissipation(neighboring, areaMatrix(:,1));
sumPollutions=getSumPollutions(carMatrix(:,[11,2,12,3]));
areaDot=zeros(9,5);
for i = 1:9
    areaDot(i,[1,2])=handleArea(dissipations(i,:),areaMatrix(i,:),sumPollutions(i,:),weather);
end
areaDot=reshape(areaDot,45,1);

carDot = zeros(length(cars)/18,18);

for i =1:length(cars)/18
   carDot(i,:) = handleCar(carMatrix(i,:),areaMatrix(:,4),areaMatrix(:,5));
end

carDot = reshape(carDot,length(cars),1);


xdot = [areaDot;carDot];
end
